simulink model "testemplanner_cs"  (R2023a)
settings: Solver=ode5  StartTime=0.0  StopTime=60  FixedStep=1/1000  RelTol=1e-3
PreLoadFcn:
  | mbxruntime.callbacks.PreLoadFcn(bdroot);
PostLoadFcn:
  | mbxruntime.callbacks.PostLoadFcn(bdroot);
InitFcn:
  | mbxruntime.callbacks.InitFcn(bdroot);
StartFcn:
  | mbxruntime.callbacks.StartFcn(bdroot);
StopFcn:
  | mbxruntime.callbacks.StopFcn(bdroot);
model workspace (MAT data in the model file):
  mbox_table : object (value not decoded)
  model_closed = 0
  sim_status = 0
undefined symbols (not defined in the file): aubr, c_factor, cf, cr, DiscIntNeverNeededParam, global_path_x, global_path_y, KD_PID_distance, KD_PID_speed, KI_PID_distance, KI_PID_speed, KP_PID_distance, KP_PID_speed, la, lb, LQR_K1, LQR_K2, LQR_K3, LQR_K4, m, rack_displacement, right_wheel_ground, tablebr, vubr, vx_break_point
libraries: PreScanSimulinkLibrary x14, Solver_SF x1
(part 6 of 8)

== matlab function testemplanner_cs/Audi_A8_Sedan_1/decision&planning module1/EM Planner/Dynamic Programming&Increase DP Node/Dynamic Programming ==
  data: dp_path_s output; dp_path_l output; planning_start_s input; planning_start_l input; planning_start_dl input; obs_s_set input; obs_l_set input; row input; col input; sample_s input; sample_l input; w_dl_smooth_cost input; w_ddl_smooth_cost input; w_dddl_smooth_cost input; w_reference_cost input; w_collision_cost input
function [dp_path_s, dp_path_l] = fcn(planning_start_s, planning_start_l, planning_start_dl, obs_s_set,...
    obs_l_set, row, col, sample_s, sample_l, w_dl_smooth_cost, w_ddl_smooth_cost, w_dddl_smooth_cost, w_reference_cost, w_collision_cost)

%该函数是动态规划（决策算法）的主函数
%要写的太多了，想起什么写什么吧

%node_cost(i,j)为起点到当前节点的最小代价
%每一列中有一个最小的数，代表起点到该列的最小代价
%最后一列的最小数即为起点到最后一列的最小代价，即为我们需要的粗解

%初始化
node_cost = ones(row, col)*inf;
point_s = zeros(row,col);
point_l = zeros(row, col);
point_dl = zeros(row, col);
point_ddl = zeros(row, col);

%下面会计算起点到第一列的最小代价
for i = 1:row
    
    %对于某奇数行的点阵，例如row=3,point_l(11)=1*sample_l,point_l(31)=-1*sample_l
    point_s(i, 1) = planning_start_s+sample_s;
    point_l(i, 1) = ((row+1)/2-i)*sample_l;

    start_cost = CalStartCost(planning_start_s, planning_start_l, w_dl_smooth_cost...
    , w_ddl_smooth_cost, w_dddl_smooth_cost, sample_s, obs_s_set, planning_start_s+sample_s, ...
    i, w_reference_cost, obs_l_set, w_collision_cost, planning_start_dl, row, sample_l);    

    %计算第一列每个点到起点的node_cost
    node_cost(i, 1) = start_cost;

end

%下面将计算从第二列开始每一个点的node_cost
%定义pre_node_index，用来记录当前点的最优路径下，上一个点所对应的行号（列号为当前点-1，无需记录）
%例如有如下点阵,最优路径为（33）<（22）<(11)
%...
%...
%...
%则pre_node_index(33)=2,pre_node_index(22)=1,pre_node_index(11)=0(行数0表示起点)

%初始化pre_node_index矩阵，其值均设为0
pre_node_index = zeros(row, col);

%下面是动态规划的主函数(从第二列开始)
for j = 2:col
    for i = 1:row
        %例如node_cost(1,j)=node_cost(i,j-1)+neighbor_cost(i,j-1)>(1,j)
        %下面要写遍历算法，记录下第二列每个点的node_cost（遍历的是第一列每个点的代价）及pre_node_index
        current_point_s = planning_start_s+j*sample_s;
        current_point_l = ((row+1)/2-i)*sample_l;
        for k = 1:row
            %调用计算相邻点代价的函数
            start_point_s = planning_start_s+(j-1)*sample_s;
            start_point_l = ((row+1)/2-k)*sample_l;
            neighbor_cost = CalcNeighborCost(start_point_s, start_point_l, w_dl_smooth_cost...
            , w_ddl_smooth_cost, w_dddl_smooth_cost, sample_s, obs_s_set, current_point_s, ...
            current_point_l, w_reference_cost, obs_l_set, w_collision_cost);
            temp_node_cost = node_cost(k, j-1)+neighbor_cost;
            if temp_node_cost < node_cost(i, j)
                node_cost(i, j) = temp_node_cost;
                pre_node_index(i, j) = k;
            end

        end
    end
end

%到这里就写完了动态规划的大部分内容，可以遍历最后一列得到最小代价，以及此路径对应的上一列的行数
%反向递推到第一列就获得了动态规划的结果（粗解）

%row_line（i)为粗解的第i列所对应的行号
row_line = zeros(col, 1);
min_node_cost = inf;

for i = 1:row
    if node_cost(i, col) < min_node_cost
        min_node_cost = node_cost(i, col);
        row_line(col) = i;
    end
end

%映射最优点的pre_node_index,也就是上一列的行号
for j = col-1:-1:1
    row_line(j) = pre_node_index(row_line(j+1), j+1);
end

%将输出初始化，由于事先不知道横纵向的采样数，因此要做缓冲
dp_path_s = ones(15, 1)*-1;
dp_path_l = ones(15, 1)*-1;
for i = 1:col
    dp_path_s(i) = planning_start_s+i*sample_s;
    dp_path_l(i) = ((row+1)/2-row_line(i))*sample_l;
end
end

%这里定义计算临近点代价的函数，与第一列到起点代价的计算很接近，注意起始点dl,ddl不同...
    function neighbor_cost = CalcNeighborCost(start_point_s, start_point_l, w_dl_smooth_cost...
            , w_ddl_smooth_cost, w_dddl_smooth_cost, sample_s, obs_s_set, current_point_s, ...
            current_point_l, w_reference_cost, obs_l_set, w_collision_cost)

        %用五次多项式连接起点到刚刚生成的点
        %五次多项式有六个边界条件
        start_l = start_point_l;
        start_dl = 0;
        start_ddl = 0;
        end_l = current_point_l;
        end_dl = 0;
        end_ddl = 0;
        start_s = start_point_s;
        end_s = current_point_s;
        %下面定义根据起点中点的六个边界条件计算五次多项式
        cofficient = CalcPathFiveCoff(start_s, end_s, start_l, start_dl, start_ddl, end_l, end_dl, end_ddl);
    
        %已经将起点和第一列的第一个点用五次多项式连接起来，将六个系数提取出来
        a0 = cofficient(1);
        a1 = cofficient(2);
        a2 = cofficient(3);
        a3 = cofficient(4);
        a4 = cofficient(5);
        a5 = cofficient(6);
    
        %在曲线上均匀提取十个采样点
        sample_point_s = zeros(10,1);
        sample_point_l = zeros(10,1);
        sample_point_dl = zeros(10,1);
        sample_point_ddl = zeros(10,1);
        sample_point_dddl = zeros(10,1);
        for m = 1:10
            sample_point_s(m) = start_s+(m-1)*sample_s/10; %（第一个）采样点的s
        end
    
        %五次多项式为：a0+a1*s+a2*s^2+a3*s^3+a4*s^4+a5*s^5,根据采样点s计算l,dl,ddl,dddl
        sample_point_l = a0+a1*sample_point_s+a2*sample_point_s.^2+a3*sample_point_s.^3+a4*sample_point_s.^4+...
            a5*sample_point_s.^5;
        sample_point_dl = a1+2*a2*sample_point_s+3*a3*sample_point_s.^2+4*a4*sample_point_s.^3+5*a5*sample_point_s.^4;
        sample_point_ddl = 2*a2+6*a3*sample_point_s+12*a4*sample_point_s.^2+20*a5*sample_point_s.^3;
        sample_point_dddl = 6*a3+24*a4*sample_point_s+60*a5*sample_point_s.^2;
        
        %计算平滑代价、参考线距离代价
        smooth_cost = w_dl_smooth_cost*(sample_point_dl'*sample_point_dl)+w_ddl_smooth_cost*(sample_point_ddl'*sample_point_ddl)...
            +w_dddl_smooth_cost*(sample_point_dddl'*sample_point_dddl);
        reference_cost = w_reference_cost*(sample_point_l'*sample_point_l);
    
        %定义障碍物代价函数,遍历每个障碍物计算代价做累加
        collision_cost = 0;
        for n = 1:length(obs_s_set)
            if isnan(obs_s_set(n))
                break;
            end
            d_long = sample_point_s-ones(10, 1)*obs_s_set(n);
            d_later = sample_point_l-ones(10, 1)*obs_l_set(n);
            square_d = d_long.^2+d_later.^2;
            collision_cost_once = CalcCollCost(w_collision_cost, square_d);
            collision_cost = collision_cost+collision_cost_once; 
            % %判断障碍物跟轨迹的位置关系
            v1 = [sample_point_s(end)-sample_point_s(1);
                  sample_point_l(end)-sample_point_l(1)];
            v2 = [obs_s_set(n)-sample_point_s(1);
                  obs_l_set(n)-sample_point_l(1)];
            flag = v1(1)*v2(2)-v1(2)*v2(1);
            if flag < 0 && collision_cost > 0
                collision_cost = collision_cost-3000;
            end
        end
    
        %计算相邻两点的neighbor_cost
        neighbor_cost = smooth_cost+reference_cost+collision_cost;

    end

%在这里定义碰撞代价函数
    function collision_cost = CalcCollCost(w_collision_cost, square_d)

        
        %我们认为障碍物与自车距离大于4米时无代价，3<距离<4时代价为1000/square_distance,距离<3时代价为w_collision_cost
        %其中square_distance为ds^2+dl^2,也就是距离的平方
        % ds = (obs_s*ones(10,1)-sample_point_s);
        % dl = (obs_l*ones(10,1)-sample_point_l);
        % square_distance = ds.^2+dl.^2;
        % collision_cost = 0; 
        % for q = 1:length(square_d)
        %     if square_d(q) > 9 && square_d(q) < 16
        %         collision_cost = collision_cost+1000/square_d(q);
        %     elseif square_d(q) < 9
        %         collision_cost = collision_cost+w_collision_cost;        
        %     end
        % end

        min_d = inf;
        for i = 1:length(square_d)
            if square_d(i) < min_d
                min_d = square_d(i);
            end
        end

        collision_cost = w_collision_cost*10^(-min_d/3);

    end

%在这里定义计算五次多项式的函数
function Path_Five_Coff = CalcPathFiveCoff(start_s, end_s, start_l, start_dl, start_ddl, end_l, end_dl, end_ddl)
    %l = a0+a1*s+a2*s^2+a3*s^3+a4*s^4+a5*s^5
    %dl = a1+2*a2*s+3*a3*s^2+4*a4*s^3+5*a5*s^4
    %ddl = 2*a2+6*a3*s+12*a4*s^2+20*a5*s^3
    
    A = [1, start_s, start_s^2, start_s^3, start_s^4, start_s^5;
         0, 1, 2*start_s, 3*start_s^2, 4*start_s^3, 5*start_s^4;
         0, 0, 2, 6*start_s, 12*start_s^2, 20*start_s^3;
         1, end_s, end_s^2, end_s^3, end_s^4, end_s^5;
         0, 1, 2*end_s, 3*end_s^2, 4*end_s^3, 5*end_s^4;
         0, 0, 2, 6*end_s, 12*end_s^2, 20*end_s^3];

    B = [start_l;
         start_dl;
         start_ddl;
         end_l;
         end_dl;
         end_ddl];

    Path_Five_Coff = A\B;
end

function start_cost = CalStartCost(start_point_s, start_point_l, w_dl_smooth_cost , w_ddl_smooth_cost, w_dddl_smooth_cost...
    , sample_s, obs_s_set, current_point_s, current_point_l, w_reference_cost, obs_l_set, w_collision_cost, start_point_dl...
    , row, sample_l)

%用五次多项式连接起点到刚刚生成的点
    %五次多项式有六个边界条件
    start_l = start_point_l;
    start_dl = start_point_dl;
    start_ddl = 0;
    end_l = ((row+1)/2-current_point_l)*sample_l;
    end_dl = 0;
    end_ddl = 0;
    start_s = start_point_s;
    end_s = current_point_s;
    %下面定义根据起点中点的六个边界条件计算五次多项式
    cofficient = CalcPathFiveCoff(start_s, end_s, start_l, start_dl, start_ddl, end_l, end_dl, end_ddl);

    %已经将起点和第一列的第一个点用五次多项式连接起来，将六个系数提取出来
    a0 = cofficient(1);
    a1 = cofficient(2);
    a2 = cofficient(3);
    a3 = cofficient(4);
    a4 = cofficient(5);
    a5 = cofficient(6);

    %在曲线上均匀提取十个采样点
    sample_point_s = zeros(10,1);
    sample_point_l = zeros(10,1);
    sample_point_dl = zeros(10,1);
    sample_point_ddl = zeros(10,1);
    sample_point_dddl = zeros(10,1);
    for j = 1:10
        sample_point_s(j) = start_s+(j-1)*sample_s/10; %（第一个）采样点的s
    end

    %五次多项式为：a0+a1*s+a2*s^2+a3*s^3+a4*s^4+a5*s^5,根据采样点s计算l,dl,ddl,dddl
    sample_point_l = a0+a1*sample_point_s+a2*sample_point_s.^2+a3*sample_point_s.^3+a4*sample_point_s.^4+...
        a5*sample_point_s.^5;
    sample_point_dl = a1+2*a2*sample_point_s+3*a3*sample_point_s.^2+4*a4*sample_point_s.^3+5*a5*sample_point_s.^4;
    sample_point_ddl = 2*a2+6*a3*sample_point_s+12*a4*sample_point_s.^2+20*a5*sample_point_s.^3;
    sample_point_dddl = 6*a3+24*a4*sample_point_s+60*a5*sample_point_s.^2;
    
    %计算平滑代价、参考线距离代价
    smooth_cost = w_dl_smooth_cost*(sample_point_dl'*sample_point_dl)+w_ddl_smooth_cost*(sample_point_ddl'*sample_point_ddl)...
        +w_dddl_smooth_cost*(sample_point_dddl'*sample_point_dddl);
    reference_cost = w_reference_cost*(sample_point_l'*sample_point_l);

    %定义障碍物代价函数,遍历每个障碍物计算代价做累加
    collision_cost = 0;
    for k = 1:length(obs_s_set)
        if isnan(obs_s_set(k))
            break;
        end
            d_long = sample_point_s-ones(10, 1)*obs_s_set(k);
            d_later = sample_point_l-ones(10, 1)*obs_l_set(k);
            square_d = d_long.^2+d_later.^2;
            collision_cost_once = CalcCollCost(w_collision_cost, square_d);
            collision_cost = collision_cost+collision_cost_once; 
            % %判断障碍物跟轨迹的位置关系
            v1 = [sample_point_s(end)-sample_point_s(1);
                  sample_point_l(end)-sample_point_l(1)];
            v2 = [obs_s_set(k)-sample_point_s(1);
                  obs_l_set(k)-sample_point_l(1)];
            flag = v1(1)*v2(2)-v1(2)*v2(1);
            if flag < 0 && collision_cost > 0
                collision_cost = collision_cost-10000;
            end
    end

    start_cost = smooth_cost+reference_cost+collision_cost;

end

== matlab function testemplanner_cs/Audi_A8_Sedan_1/decision&planning module1/EM Planner/Dynamic Programming&Increase DP Node/MATLAB Function ==
  data: dp_path_s_init input; dp_path_s_final output; dp_path_l_init input; plan_start_s input; plan_start_l input; plan_start_dl input; plan_start_ddl input; dp_path_l_final output; dp_path_dl_final output; dp_path_ddl_final output
function [dp_path_s_final, dp_path_l_final, dp_path_dl_final, dp_path_ddl_final] = fcn(dp_path_s_init, dp_path_l_init, plan_start_s, plan_start_l...
    , plan_start_dl, plan_start_ddl)

%dp_path_x_init中s方向每隔10m采样一个点，并不是一条密集连续的轨迹，要对轨迹增密
%我们并不知道s方向的采样间隔是多少（可能是10，12，15...），但传感器能探测到的范围大概为60m
%假设ds=1，即每隔1m采样一个点，设置最终轨迹的大小为60，即最多存储60个点（设置缓冲）

ds = 1;
dp_path_s_final = ones(60, 1)*nan;
dp_path_l_final = ones(60, 1)*nan;
dp_path_dl_final = ones(60, 1)*nan;
dp_path_ddl_final = ones(60, 1)*nan;

%设置动态数组用来存储采样点
l_temp = [];
dl_temp = [];
ddl_temp = [];

%设置五次多项式起点
start_s = plan_start_s;
start_l = plan_start_l;
start_dl = plan_start_dl;
start_ddl = plan_start_ddl;

for i = 1:length(dp_path_s_init)
    
    %声明一个动态数组存放采样点的s
    s_cur = [];

    if dp_path_s_init(i) == -1
        break;
    end
    
    %设置内层循环，终点是final_path_s_init(i)
    for j = 1:10000
        s_node = start_s+(j-1)*ds;
        if s_node < dp_path_s_init(i)
            s_cur = [s_cur, s_node];
        else
            break;
        end
    end

    %设置五次多项式终点
    end_s = dp_path_s_init(i);
    end_l = dp_path_l_init(i);
    end_dl = 0;
    end_ddl = 0;
    
    %调用五次多项式函数求解s_cur所对应的l
    Coff = CalcPathFiveCoff(start_s, end_s, start_l, start_dl, start_ddl, end_l, end_dl, end_ddl);
    a0 = Coff(1);
    a1 = Coff(2);
    a2 = Coff(3);
    a3 = Coff(4);
    a4 = Coff(5);
    a5 = Coff(6);
    l = a0*ones(1, length(s_cur))+a1*s_cur+a2*s_cur.^2+a3*s_cur.^3+a4*s_cur.^4+a5*s_cur.^5;
    dl = a1*ones(1, length(s_cur))+2*a2*s_cur+3*a3*s_cur.^2+4*a4*s_cur.^3+5*a5*s_cur.^4;
    ddl = 2*a2*ones(1, length(s_cur))+6*a3*s_cur+12*a4*s_cur.^2+20*a5*s_cur.^3;
    l_temp = [l_temp, l];
    dl_temp = [dl_temp, dl];
    ddl_temp = [ddl_temp, ddl];

    %给s,lfinal赋值，注意l,dl,ddl是扩展的，s_cur是一次性的，每次循环最后要清零
    for k = 1:length(l_temp)
        if k == 61
            break;
        end
        dp_path_s_final(k) = plan_start_s+(k-1)*ds;
        dp_path_l_final(k) = l_temp(k);
        dp_path_dl_final(k) = dl_temp(k);
        dp_path_ddl_final(k) = ddl_temp(k);
    end
 
    %为下一次循环赋值
    start_s = end_s;
    start_l = end_l;
    start_dl = end_dl;
    start_ddl = end_ddl;
   
end

end

%在这里定义计算五次多项式的函数
function Path_Five_Coff = CalcPathFiveCoff(start_s, end_s, start_l, start_dl, start_ddl, end_l, end_dl, end_ddl)
    %l = a0+a1*s+a2*s^2+a3*s^3+a4*s^4+a5*s^5
    %dl = a1+2*a2*s+3*a3*s^2+4*a4*s^3+5*a5*s^4
    %ddl = 2*a2+6*a3*s+12*a4*s^2+20*a5*s^3
    
    A = [1, start_s, start_s^2, start_s^3, start_s^4, start_s^5;
         0, 1, 2*start_s, 3*start_s^2, 4*start_s^3, 5*start_s^4;
         0, 0, 2, 6*start_s, 12*start_s^2, 20*start_s^3;
         1, end_s, end_s^2, end_s^3, end_s^4, end_s^5;
         0, 1, 2*end_s, 3*end_s^2, 4*end_s^3, 5*end_s^4;
         0, 0, 2, 6*end_s, 12*end_s^2, 20*end_s^3];

    B = [start_l;
         start_dl;
         start_ddl;
         end_l;
         end_dl;
         end_ddl];

    Path_Five_Coff = A\B;
end

== matlab function testemplanner_cs/Audi_A8_Sedan_1/decision&planning module1/EM Planner/Dynamic Programming&Increase DP Node/path decision with dynamic planning(dp) ==
  data: obs_s_set input; dp_path_s output; obs_l_set input; plan_start_s input; plan_start_l input; plan_start_dl input; plan_start_dll input; w_cost_collision input; w_cost_smooth_dl input; w_cost_smooth_ddl input; w_cost_smooth_dddl input; w_cost_ref input; row input; col input; sample_s input; sample_l input; dp_path_l output
function [dp_path_s,dp_path_l] = fcn(obs_s_set,obs_l_set,plan_start_s,plan_start_l,plan_start_dl,...
    plan_start_dll,w_cost_collision,w_cost_smooth_dl,w_cost_smooth_ddl,w_cost_smooth_dddl,w_cost_ref,row,col,sample_s,sample_l)
%该函数为路径决策算法动态规划的主函数
% 输入：obs s l set 筛选后的障碍物sl信息
%       plan_start s l dl ddl 规划起点信息
%       w_cost_obs,w_cost_smooth_dl,w_cost_smooth_ddl,w_cost_smooth_dddl,w_cost_ref动态规划代价权重
%       row col 动态规划采样点的行数和列数(row必须是奇数，col必须是6)
%       sample_s,sample_l 采样的s l 长度
% 输出：dp_path_l,dp_path_s 动态规划的路径sl,此路径不包含规划起点  

%动态规划最优的数据结构是结构体矩阵，但是simulink不支持结构体矩阵，所以动态规划算法写的相对难以理解

%声明二维矩阵变量node_cost，node_cost(i,j)表示从起点出发，到行i列j节点的最小代价为node_cost(i,j)
node_cost = ones(row,col)*inf;%初始化为无穷大

%声明二维矩阵变量pre_node_index pre_node_index(i,j)表示从起点到行i列j的节点的最优路径中前一个节点的行号为
%pre_node_index(i,j)
%例：比如一条最优路径为 起点 -> node(1,1) -> node(2,2) -> node(3,3)
%则pre_node_index(3,3) = 2 (最优路径的前一个节点是node(2,2) 取它的行号）
%  pre_node_index(2,2) = 1 (最优路径的前一个节点是node(1,1) 取它的行号）
%  pre_node_index(1,1) = 0 (起点的行号默认是0)

% 其实pre_node_index就是当找到最小代价的路径后从终点到起点反向选择出最优路径的
%如果用结构体矩阵完全没有必要弄得这么麻烦，但是simulink不支持
pre_node_index = zeros(row,col);%初始化，所有节点的上个最优节点的行号都是0，也就是起点

%先计算从起点到第一列的cost
for i = 1:row
    node_cost(i,1) = CalcStartCost(plan_start_s,plan_start_l,plan_start_dl,...
    plan_start_dll,i,sample_s,sample_l,w_cost_collision,w_cost_smooth_dl,...
    w_cost_smooth_ddl,w_cost_smooth_dddl,w_cost_ref,obs_s_set,obs_l_set,row);
end
% 动态规划主函数，从第二列开始
for j = 2:col
    for i = 1:row
        %计算当前node(i,j)的s l
        cur_node_s = plan_start_s + j * sample_s;
        cur_node_l = ((row + 1)/2 - i) * sample_l;
        %遍历前一列的节点
        for k = 1:row
            %计算前一列节点的s l
            pre_node_s = plan_start_s + (j - 1) * sample_s;
            pre_node_l = ((row + 1)/2 - k) * sample_l;
            cost_neighbour = CalcNeighbourCost(pre_node_s,pre_node_l,cur_node_s,cur_node_l,w_cost_collision,...
    w_cost_smooth_dl,w_cost_smooth_ddl,w_cost_smooth_dddl,w_cost_ref,obs_s_set,obs_l_set);
            %起点到上一个节点的最小代价为node_cost(k,j-1)
            pre_min_cost = node_cost(k,j-1);
            %起点到node_cost(i,j)的最小代价 为node_cost(k,j-1)
            %再加上node(k,j-1)到node(i,j)的代价 (k = 1,2,3,4...row) 中最小的
            cost_temp = pre_min_cost + cost_neighbour;
            if cost_temp < node_cost(i,j)
                node_cost(i,j) = cost_temp;
                %把最优路径上一列节点的行号记录下来
                pre_node_index(i,j) = k;
            end
        end      
    end
end
%找到node_cost最后一列中，cost最小的，记代价最小的行号为index
index = 0;
min_cost = inf;
for i = 1:row
    if node_cost(i,end) < min_cost
        min_cost = node_cost(i,end);
        index = i;
    end
end
%动态规划最优路径初始化
dp_node_list_row = zeros(col,1);
%从后往前逆推
cur_index = index;
for i = 1:col
    %记录cur_index前面节点的行号
    pre_index = pre_node_index(cur_index,end - i + 1);
    %把cur_index放到dp_node_list_row对应的位置
    dp_node_list_row(col - i + 1) = cur_index;
    %再把pre_index 赋给 cur_index 进行下一步递推
    cur_index = pre_index;
end
% 输出初始化，由于事先不知道横纵向的采样列数，因此需要做缓冲
dp_path_s = ones(15,1)*-1;
dp_path_l = ones(15,1)*-1;
for i = 1:col
    dp_path_s(i) = plan_start_s + i * sample_s;
    dp_path_l(i) = ((row + 1) / 2 - dp_node_list_row(i)) * sample_l;
end








end
function cost = CalcNeighbourCost(pre_node_s,pre_node_l,cur_node_s,cur_node_l,w_cost_collision,...
    w_cost_smooth_dl,w_cost_smooth_ddl,w_cost_smooth_dddl,w_cost_ref,obs_s_set,obs_l_set)
% 该函数将计算相邻两个节点之间的cost
  
    start_l = pre_node_l;
    start_dl = 0;
    start_ddl = 0;
    end_l = cur_node_l;
    end_dl = 0;
    end_ddl = 0;
    start_s = pre_node_s;
    end_s = cur_node_s;
    coeff = CalcQuinticCoeffient(start_l,start_dl,start_ddl,end_l,end_dl,end_ddl,start_s,end_s);
    a0 = coeff(1);
    a1 = coeff(2);
    a2 = coeff(3);
    a3 = coeff(4);
    a4 = coeff(5);
    a5 = coeff(6);
    % 取10个点计算cost
    ds = zeros(10,1);
    l = zeros(10,1);
    dl = zeros(10,1);
    ddl = zeros(10,1);
    dddl = zeros(10,1);
    for i = 1:10
        ds(i) = start_s + (i-1)*(end_s - start_s)/10;
    end
    l = a0 * ones(10,1) + a1 * ds + a2 * ds.^2 + a3 * ds.^3 + a4 * ds.^4 + a5 * ds.^5;
    dl = a1 * ones(10,1) + 2 * a2 * ds + 3 * a3 * ds.^2 + 4 * a4 * ds.^3 + 5 * a5 * ds.^4;
    ddl = 2 * a2 * ones(10,1) + 6 * a3 * ds + 12 * a4 * ds.^2 + 20 * a5 * ds.^3;
    dddl = 6 * ones(10,1) * a3 + 24 * a4 * ds + 60 * a5 * ds.^2;
    cost_smooth = w_cost_smooth_dl * (dl' * dl) + w_cost_smooth_ddl * (ddl' * ddl) + w_cost_smooth_dddl * (dddl' * dddl);
    for i = 1:length(ddl)
        if abs(ddl(i))> 0.5 || abs(atan(dl(i))) > 0.4*pi
            cost_smooth = cost_smooth + 1e7;
            break;
        end
    end
    cost_ref = w_cost_ref * (l' * l);
    cost_collision = 0;
    for i = 1:length(obs_s_set)
        if isnan(obs_s_set(i))
            break;
        end
        dlon = ones(10,1) * obs_s_set(i) - ds;
        dlat = ones(10,1) * obs_l_set(i) - l;
        %这里做了非常简化的质点模型，认为障碍物就是一个点
        square_d = dlon.^2 + dlat.^2;
        cost_collision_once = CalcObsCost(w_cost_collision,square_d);
        cost_collision = cost_collision + cost_collision_once;
        % 判断障碍物的左右
        v1 = [ds(end);l(end)] - [ds(1);l(1)];
        v2 = [obs_s_set(i);obs_l_set(i)] - [ds(1);l(1)];
        flag = v1(1)*v2(2) - v1(2)*v2(1);
        if flag < 0 && cost_collision > 0
            cost_collision = cost_collision - 1000;
        end
    end
    
    cost = cost_collision + cost_smooth + cost_ref;


end


function cost = CalcStartCost(begin_s,begin_l,begin_dl,begin_ddl,cur_node_row,sample_s,sample_l,w_cost_collision,...
    w_cost_smooth_dl,w_cost_smooth_ddl,w_cost_smooth_dddl,w_cost_ref,obs_s_set,obs_l_set,row)
    %该函数将计算起点到第一层的cost
    start_l = begin_l;
    start_dl = begin_dl;
    start_ddl = begin_ddl;
    %  . . .
    %  . . . row = 3 中间的行号 = (row + 1) /2 = 2
    %  . . .
    end_l = ((row + 1)/2 - cur_node_row)*sample_l;
    end_dl = 0;
    end_ddl = 0;
    start_s = begin_s;
    end_s = begin_s + sample_s;
    coeff = CalcQuinticCoeffient(start_l,start_dl,start_ddl,end_l,end_dl,end_ddl,start_s,end_s);
    a0 = coeff(1);
    a1 = coeff(2);
    a2 = coeff(3);
    a3 = coeff(4);
    a4 = coeff(5);
    a5 = coeff(6);
    % 取10个点计算cost
    ds = zeros(10,1);
    l = zeros(10,1);
    dl = zeros(10,1);
    ddl = zeros(10,1);
    dddl = zeros(10,1);
    for i = 1:10
        ds(i) = start_s + (i-1)*sample_s/10;
    end
    l = a0 * ones(10,1) + a1 * ds + a2 * ds.^2 + a3 * ds.^3 + a4 * ds.^4 + a5 * ds.^5;
    dl = a1 * ones(10,1) + 2 * a2 * ds + 3 * a3 * ds.^2 + 4 * a4 * ds.^3 + 5 * a5 * ds.^4;
    ddl = 2 * a2 * ones(10,1) + 6 * a3 * ds + 12 * a4 * ds.^2 + 20 * a5 * ds.^3;
    dddl = 6 * ones(10,1) * a3 + 24 * a4 * ds + 60 * a5 * ds.^2;
    cost_smooth = w_cost_smooth_dl * (dl' * dl) + w_cost_smooth_ddl * (ddl' * ddl) + w_cost_smooth_dddl * (dddl' * dddl);
    for i = 1:length(dl)
        if abs(ddl(i))> 0.5 || abs(atan(dl(i))) > 0.4*pi
            cost_smooth = cost_smooth + 1e7;
            break;
        end
    end
    cost_ref = w_cost_ref * (l' * l);
    cost_collision = 0;
    for i = 1:length(obs_s_set)
        if isnan(obs_s_set(i))
            break;
        end
        dlon = ones(10,1) * obs_s_set(i) - ds;
        dlat = ones(10,1) * obs_l_set(i) - l;
        %这里做了非常简化的质点模型，认为障碍物就是一个点
        square_d = dlon.^2 + dlat.^2;
        cost_collision_once = CalcObsCost(w_cost_collision,square_d);
        cost_collision = cost_collision + cost_collision_once;
        % 判断障碍物的左右
        v1 = [ds(end);l(end)] - [ds(1);l(1)];
        v2 = [obs_s_set(i);obs_l_set(i)] - [ds(1);l(1)];
        flag = v1(1)*v2(2) - v1(2)*v2(1);
        if flag < 0 && cost_collision > 0
            cost_collision = cost_collision - 1000;
        end
    end
    
    cost = cost_collision + cost_smooth + cost_ref;
        
end

function obs_cost = CalcObsCost(w_cost_collision,square_d)
%该函数将计算障碍物的距离代价
% 暂定超过4米的cost为0 在4到3米的cost为1000/squard_d,在小于3米的cost为w_cost_collision
%   cost = 0;
%   for i = 1:length(square_d)
%       if (square_d(i) < 16 && square_d(i) > 9) 
%           cost = cost + 500/square_d(i);
%       elseif (square_d(i) <= 9)
%           cost = cost + w_cost_collision;
%       end
%   end
%   obs_cost = cost;
min_d = inf;
for i = 1:length(square_d)
    min_d = min(min_d,square_d(i));
end
    obs_cost = w_cost_collision * 10^(-min_d/3);
end

function coeff = CalcQuinticCoeffient(start_l,start_dl,start_ddl,end_l,end_dl,end_ddl,start_s,end_s)
    % l = a0 + a1*s + a2*s^2 + a3*s^3 + a4*s^4 + a5*s^5
    % l' = a1 + 2 * a2 * s + 3 * a3 * s^2 + 4 * a4 * s^3 + 5 * a5 * s^4
    % l'' = 2 * a2 + 6 * a3 * s + 12 * a4 * s^2 + 20 * a5 * s^3
    start_s2 = start_s * start_s;
    start_s3 = start_s2 * start_s;
    start_s4 = start_s3 * start_s;
    start_s5 = start_s4 * start_s;
    end_s2 = end_s * end_s;
    end_s3 = end_s2 * end_s;
    end_s4 = end_s3 * end_s;
    end_s5 = end_s4 * end_s;
    A = [1,start_s, start_s2,     start_s3,     start_s4,      start_s5;
         0 1,       2 * start_s,  3 * start_s2, 4 * start_s3,  5 * start_s4;
         0 0,       2,            6 * start_s,  12 * start_s2, 20 * start_s3;
         1,end_s, end_s2,     end_s3,     end_s4,      end_s5;
         0,1,     2 * end_s,  3 * end_s2, 4 * end_s3,  5 * end_s4;
         0,0,     2,          6 * end_s,  12 * end_s2, 20 * end_s3;];
    B = [start_l;
         start_dl;
         start_ddl;
         end_l;
         end_dl;
         end_ddl;];
     coeff = A \ B;
    
end

== matlab function testemplanner_cs/Audi_A8_Sedan_1/decision&planning module1/EM Planner/Dynamic Programming&Increase DP Node/path decision with dynamic planning(dp)1 ==
  data: obs_s_set input; dp_path_s output; obs_l_set input; plan_start_s input; plan_start_l input; plan_start_dl input; plan_start_dll input; w_cost_collision input; w_cost_smooth_dl input; w_cost_smooth_ddl input; w_cost_smooth_dddl input; w_cost_ref input; row input; col input; sample_s input; sample_l input; dp_path_l output
function [dp_path_s,dp_path_l] = fcn(obs_s_set,obs_l_set,plan_start_s,plan_start_l,plan_start_dl,...
    plan_start_dll,w_cost_collision,w_cost_smooth_dl,w_cost_smooth_ddl,w_cost_smooth_dddl,w_cost_ref,row,col,sample_s,sample_l)
%该函数为路径决策算法动态规划的主函数
% 输入：obs s l set 筛选后的障碍物sl信息
%       plan_start s l dl ddl 规划起点信息
%       w_cost_obs,w_cost_smooth_dl,w_cost_smooth_ddl,w_cost_smooth_dddl,w_cost_ref动态规划代价权重
%       row col 动态规划采样点的行数和列数(row必须是奇数，col必须是6)
%       sample_s,sample_l 采样的s l 长度
% 输出：dp_path_l,dp_path_s 动态规划的路径sl,此路径不包含规划起点  

%动态规划最优的数据结构是结构体矩阵，但是simulink不支持结构体矩阵，所以动态规划算法写的相对难以理解

%声明二维矩阵变量node_cost，node_cost(i,j)表示从起点出发，到行i列j节点的最小代价为node_cost(i,j)
node_cost = ones(row,col)*inf;%初始化为无穷大

%声明二维矩阵变量pre_node_index pre_node_index(i,j)表示从起点到行i列j的节点的最优路径中前一个节点的行号为
%pre_node_index(i,j)
%例：比如一条最优路径为 起点 -> node(1,1) -> node(2,2) -> node(3,3)
%则pre_node_index(3,3) = 2 (最优路径的前一个节点是node(2,2) 取它的行号）
%  pre_node_index(2,2) = 1 (最优路径的前一个节点是node(1,1) 取它的行号）
%  pre_node_index(1,1) = 0 (起点的行号默认是0)

% 其实pre_node_index就是当找到最小代价的路径后从终点到起点反向选择出最优路径的
%如果用结构体矩阵完全没有必要弄得这么麻烦，但是simulink不支持
pre_node_index = zeros(row,col);%初始化，所有节点的上个最优节点的行号都是0，也就是起点

%先计算从起点到第一列的cost
for i = 1:row
    node_cost(i,1) = CalcStartCost(plan_start_s,plan_start_l,plan_start_dl,...
    plan_start_dll,i,sample_s,sample_l,w_cost_collision,w_cost_smooth_dl,...
    w_cost_smooth_ddl,w_cost_smooth_dddl,w_cost_ref,obs_s_set,obs_l_set,row);
end
% 动态规划主函数，从第二列开始
for j = 2:col
    for i = 1:row
        %计算当前node(i,j)的s l
        cur_node_s = plan_start_s + j * sample_s;
        cur_node_l = ((row + 1)/2 - i) * sample_l;
        %遍历前一列的节点
        for k = 1:row
            %计算前一列节点的s l
            pre_node_s = plan_start_s + (j - 1) * sample_s;
            pre_node_l = ((row + 1)/2 - k) * sample_l;
            cost_neighbour = CalcNeighbourCost(pre_node_s,pre_node_l,cur_node_s,cur_node_l,w_cost_collision,...
    w_cost_smooth_dl,w_cost_smooth_ddl,w_cost_smooth_dddl,w_cost_ref,obs_s_set,obs_l_set);
            %起点到上一个节点的最小代价为node_cost(k,j-1)
            pre_min_cost = node_cost(k,j-1);
            %起点到node_cost(i,j)的最小代价 为node_cost(k,j-1)
            %再加上node(k,j-1)到node(i,j)的代价 (k = 1,2,3,4...row) 中最小的
            cost_temp = pre_min_cost + cost_neighbour;
            if cost_temp < node_cost(i,j)
                node_cost(i,j) = cost_temp;
                %把最优路径上一列节点的行号记录下来
                pre_node_index(i,j) = k;
            end
        end      
    end
end
%找到node_cost最后一列中，cost最小的，记代价最小的行号为index
index = 0;
min_cost = inf;
for i = 1:row
    if node_cost(i,end) < min_cost
        min_cost = node_cost(i,end);
        index = i;
    end
end
%动态规划最优路径初始化
dp_node_list_row = zeros(col,1);
%从后往前逆推
cur_index = index;
for i = 1:col
    %记录cur_index前面节点的行号
    pre_index = pre_node_index(cur_index,end - i + 1);
    %把cur_index放到dp_node_list_row对应的位置
    dp_node_list_row(col - i + 1) = cur_index;
    %再把pre_index 赋给 cur_index 进行下一步递推
    cur_index = pre_index;
end
% 输出初始化，由于事先不知道横纵向的采样列数，因此需要做缓冲
dp_path_s = ones(15,1)*-1;
dp_path_l = ones(15,1)*-1;
for i = 1:col
    dp_path_s(i) = plan_start_s + i * sample_s;
    dp_path_l(i) = ((row + 1) / 2 - dp_node_list_row(i)) * sample_l;
end








end
function cost = CalcNeighbourCost(pre_node_s,pre_node_l,cur_node_s,cur_node_l,w_cost_collision,...
    w_cost_smooth_dl,w_cost_smooth_ddl,w_cost_smooth_dddl,w_cost_ref,obs_s_set,obs_l_set)
% 该函数将计算相邻两个节点之间的cost
  
    start_l = pre_node_l;
    start_dl = 0;
    start_ddl = 0;
    end_l = cur_node_l;
    end_dl = 0;
    end_ddl = 0;
    start_s = pre_node_s;
    end_s = cur_node_s;
    coeff = CalcQuinticCoeffient(start_l,start_dl,start_ddl,end_l,end_dl,end_ddl,start_s,end_s);
    a0 = coeff(1);
    a1 = coeff(2);
    a2 = coeff(3);
    a3 = coeff(4);
    a4 = coeff(5);
    a5 = coeff(6);
    % 取10个点计算cost
    ds = zeros(10,1);
    l = zeros(10,1);
    dl = zeros(10,1);
    ddl = zeros(10,1);
    dddl = zeros(10,1);
    for i = 1:10
        ds(i) = start_s + (i-1)*(end_s - start_s)/10;
    end
    l = a0 * ones(10,1) + a1 * ds + a2 * ds.^2 + a3 * ds.^3 + a4 * ds.^4 + a5 * ds.^5;
    dl = a1 * ones(10,1) + 2 * a2 * ds + 3 * a3 * ds.^2 + 4 * a4 * ds.^3 + 5 * a5 * ds.^4;
    ddl = 2 * a2 * ones(10,1) + 6 * a3 * ds + 12 * a4 * ds.^2 + 20 * a5 * ds.^3;
    dddl = 6 * ones(10,1) * a3 + 24 * a4 * ds + 60 * a5 * ds.^2;
    cost_smooth = w_cost_smooth_dl * (dl' * dl) + w_cost_smooth_ddl * (ddl' * ddl) + w_cost_smooth_dddl * (dddl' * dddl);
    cost_ref = w_cost_ref * (l' * l);
    cost_collision = 0;
    for i = 1:length(obs_s_set)
        if isnan(obs_s_set(i))
            break;
        end
        dlon = ones(10,1) * obs_s_set(i) - ds;
        dlat = ones(10,1) * obs_l_set(i) - l;
        %这里做了非常简化的质点模型，认为障碍物就是一个点
        square_d = dlon.^2 + dlat.^2;
        cost_collision_once = CalcObsCost(w_cost_collision,square_d);
        cost_collision = cost_collision + cost_collision_once;
    end
    cost = cost_collision + cost_smooth + cost_ref;


end


function cost = CalcStartCost(begin_s,begin_l,begin_dl,begin_ddl,cur_node_row,sample_s,sample_l,w_cost_collision,...
    w_cost_smooth_dl,w_cost_smooth_ddl,w_cost_smooth_dddl,w_cost_ref,obs_s_set,obs_l_set,row)
    %该函数将计算起点到第一层的cost
    start_l = begin_l;
    start_dl = begin_dl;
    start_ddl = begin_ddl;
    %  . . .
    %  . . . row = 3 中间的行号 = (row + 1) /2 = 2
    %  . . .
    end_l = ((row + 1)/2 - cur_node_row)*sample_l;
    end_dl = 0;
    end_ddl = 0;
    start_s = begin_s;
    end_s = begin_s + sample_s;
    coeff = CalcQuinticCoeffient(start_l,start_dl,start_ddl,end_l,end_dl,end_ddl,start_s,end_s);
    a0 = coeff(1);
    a1 = coeff(2);
    a2 = coeff(3);
    a3 = coeff(4);
    a4 = coeff(5);
    a5 = coeff(6);
    % 取10个点计算cost
    ds = zeros(10,1);
    l = zeros(10,1);
    dl = zeros(10,1);
    ddl = zeros(10,1);
    dddl = zeros(10,1);
    for i = 1:10
        ds(i) = start_s + (i-1)*sample_s/10;
    end
    l = a0 * ones(10,1) + a1 * ds + a2 * ds.^2 + a3 * ds.^3 + a4 * ds.^4 + a5 * ds.^5;
    dl = a1 * ones(10,1) + 2 * a2 * ds + 3 * a3 * ds.^2 + 4 * a4 * ds.^3 + 5 * a5 * ds.^4;
    ddl = 2 * a2 * ones(10,1) + 6 * a3 * ds + 12 * a4 * ds.^2 + 20 * a5 * ds.^3;
    dddl = 6 * ones(10,1) * a3 + 24 * a4 * ds + 60 * a5 * ds.^2;
    cost_smooth = w_cost_smooth_dl * (dl' * dl) + w_cost_smooth_ddl * (ddl' * ddl) + w_cost_smooth_dddl * (dddl' * dddl);
    cost_ref = w_cost_ref * (l' * l);
    cost_collision = 0;
    for i = 1:length(obs_s_set)
        if isnan(obs_s_set(i))
            break;
        end
        dlon = ones(10,1) * obs_s_set(i) - ds;
        dlat = ones(10,1) * obs_l_set(i) - l;
        %这里做了非常简化的质点模型，认为障碍物就是一个点
        square_d = dlon.^2 + dlat.^2;
        cost_collision_once = CalcObsCost(w_cost_collision,square_d);
        cost_collision = cost_collision + cost_collision_once;
    end
    cost = cost_collision + cost_smooth + cost_ref;
        
end

function obs_cost = CalcObsCost(w_cost_collision,square_d)
%该函数将计算障碍物的距离代价
% 暂定超过4米的cost为0 在4到3米的cost为1000/squard_d,在小于3米的cost为w_cost_collision
  cost = 0;
  for i = 1:length(square_d)
      if (square_d(i) < 16 && square_d(i) > 9) 
          cost = cost + 1000/square_d(i);
      elseif (square_d(i) < 9)
          cost = cost + w_cost_collision;
      end
  end
  obs_cost = cost;

end

function coeff = CalcQuinticCoeffient(start_l,start_dl,start_ddl,end_l,end_dl,end_ddl,start_s,end_s)
    % l = a0 + a1*s + a2*s^2 + a3*s^3 + a4*s^4 + a5*s^5
    % l' = a1 + 2 * a2 * s + 3 * a3 * s^2 + 4 * a4 * s^3 + 5 * a5 * s^4
    % l'' = 2 * a2 + 6 * a3 * s + 12 * a4 * s^2 + 20 * a5 * s^3
    start_s2 = start_s * start_s;
    start_s3 = start_s2 * start_s;
    start_s4 = start_s3 * start_s;
    start_s5 = start_s4 * start_s;
    end_s2 = end_s * end_s;
    end_s3 = end_s2 * end_s;
    end_s4 = end_s3 * end_s;
    end_s5 = end_s4 * end_s;
    A = [1,start_s, start_s2,     start_s3,     start_s4,      start_s5;
         0 1,       2 * start_s,  3 * start_s2, 4 * start_s3,  5 * start_s4;
         0 0,       2,            6 * start_s,  12 * start_s2, 20 * start_s3;
         1,end_s, end_s2,     end_s3,     end_s4,      end_s5;
         0,1,     2 * end_s,  3 * end_s2, 4 * end_s3,  5 * end_s4;
         0,0,     2,          6 * end_s,  12 * end_s2, 20 * end_s3;];
    B = [start_l;
         start_dl;
         start_ddl;
         end_l;
         end_dl;
         end_ddl;];
     coeff = A \ B;
    
end

== matlab function testemplanner_cs/Audi_A8_Sedan_1/decision&planning module1/EM Planner/Frenet2Cartesian ==
  data: s_set input; l_set input; dl_set input; ddl_set input; frenet_x input; frenet_y input; frenet_heading input; frenet_kappa input; index2s input; x_point_set output; y_point_set output; heading_point_set output; kappa_point_set output
function [x_point_set, y_point_set, heading_point_set, kappa_point_set] = fcn(s_set, l_set, dl_set, ddl_set, frenet_x, ...
    frenet_y, frenet_heading, frenet_kappa, index2s)

%该函数的作用是把自然坐标系(s,l)下的粗解转换到笛卡尔坐标系（x,y）
%不确定有多少个点需要坐标转换，要做缓冲
%frenet转cartesian的步骤是：先找到待变换点在参考线上投影点的x,y，再计算待转换点的x,y

%在index2s上遍历得到匹配点编号，用匹配点求投影点的xy...

%这里可能有bug,因为s是点的投影的弧长，而不是点的匹配点的弧长，我认为找到在参考线上索引之后可以直接得到投影点的几何信息

x_point_set = ones(600, 1)*nan;
y_point_set = ones(600, 1)*nan;
heading_point_set = ones(600, 1)*nan;
kappa_point_set = ones(600, 1)*nan; 

for i = 1:length(s_set)
    if isnan(s_set(i))
        break;
    end
    %调用函数计算投影点
    [proj_point, proj_point_x, proj_point_y, proj_point_heading, proj_point_kappa] = CalcProjPoint(index2s, s_set(i), frenet_x, frenet_y, frenet_heading, frenet_kappa);
    %根据投影点的xy计算待转换点的xy
    proj_nor = [-sin(proj_point_heading); cos(proj_point_heading)];
    point = proj_point+proj_nor*l_set(i);
    x_point_set(i) = point(1);
    y_point_set(i) = point(2);
    heading_point_set(i) = atan(dl_set(i)/(1-proj_point_kappa*l_set(i)))+proj_point_heading;
    %近似认为kr'=0
    kappa_point_set(i) = ((ddl_set(i)+proj_point_kappa*dl_set(i)*tan(heading_point_set(i)-proj_point_heading))...
        *(cos(heading_point_set(i)-proj_point_heading)^2)/(1-proj_point_kappa*l_set(i))+proj_point_kappa)*cos(heading_point_set(i)-proj_point_heading)...
        /(1-proj_point_kappa*l_set(i));

end

end

%定义计算投影点的函数
function [proj_point, proj_point_x, proj_point_y, proj_point_heading, proj_point_kappa] = CalcProjPoint(index2s, s, frenet_x, frenet_y, frenet_heading, frenet_kappa)

%先遍历找到index2s上的匹配点
match_index = 1;
while index2s(match_index) < s
    match_index = match_index+1;
end
%提取数据（按照上述做法，匹配点一定在投影点之后，感觉有bug）
match_point = [frenet_x(match_index); frenet_y(match_index)];
match_point_heading = frenet_heading(match_index);
match_point_kappa = frenet_kappa(match_index);
ds = s-index2s(match_index);
match_tor = [cos(match_point_heading); sin(match_point_heading)];
proj_point = match_point+ds*match_tor;
proj_point_x = proj_point(1);
proj_point_y = proj_point(2);
proj_point_heading = match_point_heading+ds*match_point_kappa;
proj_point_kappa = match_point_kappa;
end

== matlab function testemplanner_cs/Audi_A8_Sedan_1/decision&planning module1/EM Planner/Frenet2Cartesian task ==
  data: s_set input; x_set output; l_set input; dl_set input; ddl_set input; frenet_path_x input; frenet_path_y input; frenet_path_heading input; frenet_path_kappa input; index2s input; y_set output; heading_set output; kappa_set output
function [x_set,y_set,heading_set,kappa_set] = ...
    fcn(s_set,l_set,dl_set,ddl_set,frenet_path_x,frenet_path_y,frenet_path_heading,frenet_path_kappa,index2s)
% 通用算法 frenet转frenet
% 由于不知道有多少个(s,l)要转化成直角坐标，因此做缓冲
% 输出初始化
    x_set = ones(600,1) * nan;
    y_set = ones(600,1) * nan;
    heading_set = ones(600,1) * nan;
    kappa_set = ones(600,1) * nan;
    for i = 1:length(s_set)
        if isnan(s_set(i))
            break;
        end
        % 计算(s,l)在frenet坐标轴上的投影
        [proj_x,proj_y,proj_heading,proj_kappa] = CalcProjPoint(s_set(i),frenet_path_x,frenet_path_y,frenet_path_heading,...
    frenet_path_kappa,index2s);
        nor = [-sin(proj_heading);cos(proj_heading)];
        point = [proj_x;proj_y] + l_set(i) * nor;
        x_set(i) = point(1);
        y_set(i) = point(2);
        heading_set(i) = proj_heading + atan(dl_set(i)/(1 - proj_kappa * l_set(i)));
        % 近似认为 kappa' == 0,frenet转cartesian公式，见第一章第三节评论区的链接
        kappa_set(i) = ((ddl_set(i) + proj_kappa * dl_set(i) * tan(heading_set(i) - proj_heading)) * ...
            (cos(heading_set(i) - proj_heading)^2)/(1 - proj_kappa * l_set(i)) + proj_kappa) * ...
            cos(heading_set(i) - proj_heading)/(1 - proj_kappa * l_set(i));
         
    end

end


function [proj_x,proj_y,proj_heading,proj_kappa] = CalcProjPoint(s,frenet_path_x,frenet_path_y,frenet_path_heading,...
    frenet_path_kappa,index2s)
% 该函数将计算在frenet坐标系下，点(s,l)在frenet坐标轴的投影的直角坐标(proj_x,proj_y,proj_heading,proj_kappa)'
% 先找匹配点的编号
    match_index = 1;
    while index2s(match_index) < s
        match_index = match_index + 1;
    end
    match_point = [frenet_path_x(match_index);frenet_path_y(match_index)];
    match_point_heading = frenet_path_heading(match_index);
    match_point_kappa = frenet_path_kappa(match_index);
    ds = s - index2s(match_index);
    match_tor = [cos(match_point_heading);sin(match_point_heading)];
    proj_point = match_point + ds * match_tor;
    proj_heading = match_point_heading + ds * match_point_kappa;
    proj_kappa = match_point_kappa;
    proj_x = proj_point(1);
    proj_y = proj_point(2);   
end

== matlab function testemplanner_cs/Audi_A8_Sedan_1/decision&planning module1/EM Planner/Generate Convex Space&Quadratic Programming/MATLAB Function1 ==
  data: l_min output; l_max output; static_obs_s_set input; static_obs_l_set input; obs_length input; obs_width input; dp_path_s input; dp_path_l input
function [l_min, l_max] = fcn(static_obs_s_set, static_obs_l_set, obs_length, obs_width, ...
    dp_path_s, dp_path_l)

%该函数用来开辟凸空间。计算凸空间的上下界
%障碍物在自然坐标系的几何用世界坐标系中的近似代替
%因此，在小曲率（r>200）道路精度较高，在大曲率道路需要额外处理

%初始化输出
l_min = ones(60, 1)*-6;
l_max = ones(60, 1)*6;

for i = 1:length(static_obs_s_set)
    if isnan(static_obs_s_set(i))
        break;
    end
    %计算障碍物头尾的s
    start_s = static_obs_s_set(i)+obs_length/2;
    end_s = static_obs_s_set(i)-obs_length/2;
    %计算障碍物头尾的s在dp_path_s中对应的序号
    start_index = CalcNearIndex(dp_path_s, start_s);
    end_index = CalcNearIndex(dp_path_s, end_s);

    %打个补丁
    if start_index == 1 && end_index == 1
        %代表障碍物在自车后面，不对凸空间产生影响
        continue;
    end

    %也就是说在头尾之间的上下界需要重新赋值
    %下面判断动态规划对于障碍物是向左绕（赋值下界）还是向右绕（赋值上界）
    %用障碍物中心索引对应的动态规划结果与障碍物l坐标近似判断
    % center_index = CalcNearIndex(dp_path_s, static_obs_s_set(i));
    % l_dp = dp_path_l(center_index);

    l_dp = (dp_path_l(start_index) + dp_path_l(end_index))/2;

    if l_dp > static_obs_l_set(i)
        %向左绕
        %凸空间的下界为所有向左绕的决策中范围内已有下界和障碍物上界的最大值（仔细品代码）
        for j = end_index:start_index
            l_min(j) = max(l_min(j), static_obs_l_set(i)+obs_width/2);
        end
    else
        %向右绕
        %凸空间的上界为所有向右绕的决策中范围内已有上界和障碍物下界的最小值（仔细品代码）
        for j = end_index:start_index
            l_max(j) = min(l_max(j), static_obs_l_set(i)-obs_width/2);
        end
    end
end
end

%定义计算序号的函数
function y = CalcNearIndex(dp_path_s, s)
    %在dp_path_s中都是正数，而障碍物的s坐标可能为负
        if s <= dp_path_s(1)
            %认为障碍物在自车后面
            y = 1;
            return;
        elseif dp_path_s(end) < s
            y = 60;
            return;
        else
            index = 1;
            while dp_path_s(index) < s
                index = index+1;
            end
            %要判断一下index和index-1哪个是距离s最近的索引
            if dp_path_s(index)-s > s-dp_path_s(index-1)
                y = index-1;
            else
                y = index;
            end
        end

end

== matlab function testemplanner_cs/Audi_A8_Sedan_1/decision&planning module1/EM Planner/Generate Convex Space&Quadratic Programming/MATLAB Function2 ==
  data: qp_path_s output; w_ref_cost input; qp_path_l output; w_dl_cost input; w_ddl_cost input; w_dddl_cost input; w_centre_cost input; w_end_l_cost input; w_end_dl_cost input; w_end_ddl_cost input; d1 input; d2 input; width input; lmin input; lmax input; plan_start_l input; plan_start_dl input; plan_start_ddl input; qp_path_dl output; qp_path_ddl output; dp_path_l_final input; delta_dl_max input; delta_dl_min input; delta_ddl_max input; delta_ddl_min input; plan_start_s input; centre_line output
function [qp_path_s, qp_path_l, qp_path_dl, qp_path_ddl, centre_line] = fcn(w_ref_cost, w_dl_cost, w_ddl_cost, ...
    w_dddl_cost, w_centre_cost, w_end_l_cost, w_end_dl_cost, w_end_ddl_cost, d1, d2, width, ...
    lmin, lmax, plan_start_l, plan_start_dl, plan_start_ddl, dp_path_l_final, delta_dl_max...
    , delta_dl_min, delta_ddl_max, delta_ddl_min, plan_start_s)

%二次规划
coder.extrinsic("quadprog");

n = 20;

%初始化矩阵
Aeq = zeros((2*n-2), 3*n);
beq = zeros(2*n-2, 1);
A = zeros(8*n, 3*n);
b = zeros(8*n, 1);
Hl = zeros(3*n, n);
Hdl = zeros(3*n, n);
Hddl = zeros(3*n, n);
Hdddl = zeros(3*n, n-1);
Hel = zeros(3*n, n);
Hedl = zeros(3*n, n);
Heddl = zeros(3*n, n);

qp_path_s = zeros(n, 1);
qp_path_l =zeros(n, 1);
qp_path_dl = zeros(n, 1);
qp_path_ddl = zeros(n, 1);

ds = 3;
%等式约束：Aeq*x=beq
Aeq_sub = [1, ds, ds^2/3, -1, 0, ds^2/6;
           0, 1, ds/2, 0, -1, ds/2];

%不等式约束：Ax<=b
A_sub = [1, d1, 0;
         1, d1, 0;
         1, -d2, 0;
         1, -d2, 0;
         -1, -d1, 0;
         -1, -d1, 0;
         -1, d2, 0;
         -1, d2, 0];

%下面计算左前（右前）及左后（右后）角点的附加编号
add_front_index = ceil(d1);
add_rear_index = ceil(d2);

%不再对规划起点进行碰撞约束
for i = 2:n
    index1 = min((3*i-2+add_front_index), 60);
    index2 = max((3*i-2-add_rear_index), 1);
    %下面生成b
    b(8*i-7:8*i, 1) = [lmax(index1)-width/2;
                       lmax(index1)+width/2;
                       lmax(index2)-width/2;
                       lmax(index2)+width/2;
                       -lmin(index1)+width/2;
                       -lmin(index1)-width/2;
                       -lmin(index2)+width/2;
                       -lmin(index2)-width/2];

end

%生成Aeq
for i = 1:n-1
    Aeq(2*i-1:2*i, 3*i-2:3*i+3) = Aeq_sub;
end

%生成A
for i = 2:n
    A(8*i-7:8*i, 3*i-2:3*i) = A_sub;
end

%生成对dl及ddl的约束
A_delta_sub = [0, -1, 0, 0, 1, 0
               0, 1, 0, 0, -1, 0;
               0, 0, -1, 0, 0, 1;
               0, 0, 1, 0, 0, -1];

b_delta_sub = [delta_dl_max;
               -delta_dl_min;
               delta_ddl_max;
               -delta_ddl_min];

%生成A-delta及b_delta
A_delta = zeros(4*n-4, 3*n);
b_delta = zeros(4*n-4, 1);
for i = 1:n-1
    A_delta(4*i-3:4*i, 3*i-2:3*i+3) = A_delta_sub;
    b_delta(4*i-3:4*i, 1) = b_delta_sub;
end

%生成Hl,Hdl,Hddl
for i = 1:n
    Hl(3*i-2, i) = 1;
    Hdl(3*i-1, i) = 1;
    Hddl(3*i, i) = 1;
end

%生成Hdddl
for i = 1:n-1
    Hdddl(3*i, i) = -1;
    Hdddl(3*i+3, i) = 1;
end

%生成Hel
Hel(3*n-2, n) = 1;
Hedl(3*n-1, n) = 1;
Heddl(3*n, n) = 1;

H = w_ref_cost*(Hl*Hl')+w_dl_cost*(Hdl*Hdl')+w_ddl_cost*(Hddl*Hddl')+w_dddl_cost/ds^2*(Hdddl*Hdddl')+w_centre_cost*(Hl*Hl')...
    +w_end_l_cost*(Hel*Hel')+w_end_dl_cost*(Hedl*Hedl')+w_end_ddl_cost*(Heddl*Heddl');
% H = w_ref_cost*(Hl'*Hl)+w_dl_cost*(Hdl'*Hdl)+w_ddl_cost*(Hddl'*Hddl)+w_dddl_cost*(Hdddl'*Hdddl)+w_centre_cost*(Hl'*Hl)...
%     +w_end_l_cost*(Hel'*Hel)+w_end_dl_cost*(Hedl'*Hedl)+w_end_ddl_cost*(Heddl'*Heddl);
% H = w_ref_cost*(Hl*Hl')+w_dl_cost*(Hdl*Hdl')+w_ddl_cost*(Hddl*Hddl')+w_dddl_cost/ds^2*(Hdddl*Hdddl')+w_centre_cost*(Hl*Hl');
H = 2*H;

%定义f所必须的矩阵声明
centre_line = (lmin+lmax)/2;
% centre_line = dp_path_l_final; %防止崩溃A1
L = zeros(n, 1);
for i = 1:n
    L(i) = centre_line(3*i-2);
    if abs(L(i)) > 0.3
        L(i) = L(i)*w_centre_cost;
    end
end

f = -2*L'*Hl';
f = f';

%二次规划会优化规划起点，但规划起点是确定的，所以要添加约束
lb = ones(3*n, 1)*-inf;
ub = ones(3*n, 1)*inf;
lb(1) = plan_start_l;
lb(2) = plan_start_dl;
lb(3) = plan_start_ddl;

ub(1) = lb(1);
ub(2) = lb(2);
ub(3) = lb(3);

for i = 2:n
    lb(3*i-1) = -2;
    ub(3*i-1) = 2;
    lb(3*i) = -0.5;
    ub(3*i) = 0.5;
end

for i = 1:n
    qp_path_s(i) = plan_start_s+(i-1)*ds;
end

%优化求解
X = quadprog(H, f, [A; A_delta], [b; b_delta], Aeq, beq, lb, ub);
% X = quadprog(H, f, A, b, Aeq, beq, [], []);
%填充矩阵
for i = 1:n
    qp_path_l(i) = X(3*i-2, 1);
    qp_path_dl(i) = X(3*i-1, 1);
    qp_path_ddl(i) = X(3*i, 1);
end

== matlab function testemplanner_cs/Audi_A8_Sedan_1/control module/control main/longitudinal control double PID/MATLAB Function1 ==
  data: u input; throttle output; brake output
function [throttle,brake] = fcn(u)
    if u>=0
        throttle=u;
        brake=0;
    else
        throttle=0;
        brake=-u;
    end

== matlab function testemplanner_cs/Audi_A8_Sedan_1/decision&planning module1/EM Planner/Generate Convex Space&Quadratic Programming/MATLAB Function3 ==
  data: qp_path_s input; qp_path_s_final output; qp_path_l input; qp_path_dl input; qp_path_ddl input; qp_path_l_final output; qp_path_dl_final output; qp_path_ddl_final output
function [qp_path_s_final,qp_path_l_final, qp_path_dl_final,qp_path_ddl_final] = fcn(qp_path_s,qp_path_l,qp_path_dl,qp_path_ddl)
% 该函数将增密qp_path
n_init = 20;
% 增密的点的个数
n = 501;
% 输出初始化
qp_path_s_final = zeros(n,1);
qp_path_l_final = zeros(n,1);
qp_path_dl_final = zeros(n,1);
qp_path_ddl_final = zeros(n,1);
ds = (qp_path_s(end) - qp_path_s(1))/(n-1);
index = 1;
for i = 1:n
    x = qp_path_s(1) + (i-1) * ds;
    qp_path_s_final(i) = x;
    while x >= qp_path_s(index)
        index = index + 1;
        if index == n_init
            break;
        end
    end
    % while 循环退出的条件是x<qp_path_s(index)，所以x对应的前一个s的编号是index-1 后一个编号是index
    pre = index - 1;
    cur = index;
    % 计算前一个点的l l' l'' ds 和后一个点的 l''
    delta_s = x - qp_path_s(pre);
    l_pre = qp_path_l(pre);
    dl_pre = qp_path_dl(pre);
    ddl_pre = qp_path_ddl(pre);
    ddl_cur = qp_path_ddl(cur);
    % 分段加加速度优化 
    qp_path_l_final(i) = l_pre + dl_pre * delta_s + (1/3)* ddl_pre * delta_s^2 + (1/6) * ddl_cur * delta_s^2;
    qp_path_dl_final(i) = dl_pre + 0.5 * ddl_pre * delta_s + 0.5 * ddl_cur * delta_s;
    qp_path_ddl_final(i) = ddl_pre + (ddl_cur - ddl_pre) * delta_s/(qp_path_s(cur) - qp_path_s(pre));
    %  因为此时x的后一个编号是index 必有x < qp_path_s(index),在下一个循环中x = x + ds 也未必大于
    %  qp_path_s(index)，这样就进入不了while循环，所以index 要回退一位
    index = index - 1;   
end
